simulink model "Final_closeloop_sinus"  (R2024b)
settings: Solver=ode23s  StartTime=0.0  StopTime=150  RelTol=1e-3
libraries: slpidlib x16
(part 2 of 2)

== matlab function Final_closeloop_sinus/M-101 ==
  data: y output; u input
function y  = MX(u) 

% inputs
Q_R = u(1);     % Recycling stream
Q_M = u(2);     % Fresh media stream
C_X_M = u(3);   % Fresh biomass concentration
C_GLU_M = u(4); % Fresh glucose concentration
C_N_M = u(5);   % Fresh nitrogen concentration
C_X_S = u(6);   % Recycle biomass concentration
C_GLU_S = u(7); % Recycle glucose concentration
C_N_S = u(8);   % Recycle nitrogen concentration


% output
y=zeros(4,1);
y(1) = (C_X_S*Q_R+C_X_M*Q_M)/(Q_M+Q_R);         %C_X_F
y(2) = (C_GLU_M*Q_M+C_GLU_S*Q_R)/(Q_M+Q_R);     %C_GLU_F
y(3) = (C_N_M*Q_M+C_N_S*Q_R)/(Q_M+Q_R);         %C_N_F
y(4) = (Q_M+Q_R);                               % Q_F

== matlab function Final_closeloop_sinus/MM-501 ==
  data: y output; u input
function y  = MX(u)

% Inputs: [Q_F, C_mRNA_F, Q_G, C_LNP_G, C_ethanol_G, C_imp1_G, C_imp2_G, C_imp3_G, encapsulation_efficiency]

% Inputs
Q_F = u(1);                                      % Flow rate from Tank F (mRNA solution)
C_mRNA_F = u(2);                                 % mRNA concentration
Q_G = u(3);                                      % Flow rate from Tank G (LNP solution)
C_LNP_G = u(4);                                  % LNP concentration (Tank G)
C_ethanol_G = u(5);                              % Ethanol concentration
C_sucrose_G = u(6);                              % Sucrose concentration
C_imp1_G = u(7);                                 % Impurity 1 concentration 
C_imp2_G = u(8);                                 % Impurity 2 concentration

y = zeros(7, 1);

y(1) = (C_mRNA_F * Q_F)/(Q_F + Q_G);       % Encapsulated mRNA-LNP (assumed 100% encapsulated)
y(2) = (C_LNP_G * Q_F)/(Q_F + Q_G);       % Encapsulated LNP (assumed 100% encapsulated)
y(3) = (C_ethanol_G* Q_G) / (Q_F + Q_G);         % C_ethanol
y(4) = (C_sucrose_G* Q_G) / (Q_F + Q_G);         % C_ethanol
y(5) = (C_imp1_G * Q_G) / (Q_F + Q_G);           % C_Impurity 1
y(6) = (C_imp2_G * Q_G) / (Q_F + Q_G);           % C_Impurity 2
y(7) = (Q_F + Q_G);                                % Total flow rate

end

== matlab function Final_closeloop_sinus/NF-501 ==
  data: u input; y output
function y = NF(u)
%% parameters for nanofiltration 
% a DOW NF90 nanofiltration membrane has been chosen. This type of membrane
% has been used in pharmaceutical applications for API filtrations (title
% reference: Removal of antibiotics from a model wastewater by RO/NF membranes)
%A=0.398443840087261; %membrane surface area [m^2] 
%% parameters for nanofiltration 
%A=0.3984033;
Jw=57.90; %permeate flowrate at 8 bar pressure [l/m^2/h]
Res=Jw/8; %[l/m^2/h/bar]function y  = NN(u)


%input
C_mRNALNP_4=u(1);
C_LNP_4=u(2);
C_Ethanol_4=u(3);
C_Sucrose_4=u(4);
C_IMP1_4=u(5);
C_IMP2_4=u(6);
Q_IN=u(7);
P=u(8);
A=u(9);

tlim=1;
dim=14;
y=zeros(dim,1);


%% Rejection coefficients for different species
Rej=[0.00002*P^4 - 0.0018*P^3 + 0.0145*P^2 + 0.0849*P + 0.22248; 0.01; 0.01; 0.00002*P^4 - 0.0018*P^3 + 0.0145*P^2 + 0.0849*P + 0.22248; 0.01; 0.99];


%% Output calculations

     y(1)=A*Res*P;%permeate volumetric flowrate [l/h];(ref: Continuous purification of
    %active pharmaceutical ingredients using multistage organic solvent nanofiltration membrane cascade)
    y(2)=Q_IN-y(1); %balance on centrifugation+filtration
    

%% Species balances for retentate stream (calculated based on inflow and rejection)
    y(3)=(Q_IN*C_mRNALNP_4)/(y(2)+y(1)*(1-Rej(1)));         % mRNA-LNP concentration in retentate stream
    y(4)=(Q_IN*C_LNP_4)/(y(2)+y(1)*(1-Rej(2)));         % LNP concentration in retentate stream
    y(5)=(Q_IN*C_Ethanol_4)/(y(2)+y(1)*(1-Rej(3)));         % Ethanol concentration in retentate stream
    y(6)=(Q_IN*C_Sucrose_4)/(y(2)+y(1)*(1-Rej(4)));         % Sucrose concentration in retentate stream
    y(7)=(Q_IN*C_IMP1_4)/(y(2)+y(1)*(1-Rej(5)));            % Impurity 1 concentration in retentate stream
    y(8)=(Q_IN*C_IMP2_4)/(y(2)+y(1)*(1-Rej(6)));            % Impurity 2 concentration in retentate stream
   
 %% Species concentrations in permeate stream (calculated based on rejection)
    y(9)=y(3)*(1-Rej(1));                                   % mRNA-LNP concentration in permeate stream
    y(10)=y(4)*(1-Rej(2));                                   % LNP concentration in permeate stream
    y(11)=y(5)*(1-Rej(3));                                   % Ethanol concentration in permeate stream
    y(12)=y(6)*(1-Rej(4));                                  % Sucrose concentration in permeate stream
    y(13)=y(7)*(1-Rej(5));                                  % Impurity 1 concentration in permeate stream
    y(14)=y(8)*(1-Rej(6));                                  % Impurity 2 concentration in permeate stream
  

end

== matlab function Final_closeloop_sinus/VSP-503 ==
  data: u input size=2; y output size=2
function y  = Pump(u)

%input
Q_C=u(1);
n=u(2);


y=zeros(2,1);

% output

y(1)=Q_C;
y(2)=((-0.085*Q_C^2 - 0.0000329*Q_C*n + 0.0000155555555555556*n^2)*(997*9.81))/10^5;


end

== matlab function Final_closeloop_sinus/MATLAB Function1 ==
  data: u input; y output
function y = Formulation_medium(u)
    % Inputs
    Q = u(1);                                   % Total flow rate (L/h)
    C_mRNA = u(2);                              % Concentration of mRNA (g/L)

    % Distribution of flow rates
    Q_Ethanol = Q/3;                            % Ethanol flow (1/3 of total flow)
    Q_LNP = Q / 3;                              % LNP flow (1/3 of total flow)
    Q_Sucrose = Q*10;                            % LNP flow (1/3 of total flow)

    % Concentrations
    C_LNP = C_mRNA / 0.029;                     % LNP concentration (g/g)
    C_Sucrose = Q_Sucrose *0.1;                   % Sucrose concentration
    C_Impurities_1 = Q_Ethanol * 0.05;          % Impurity 1: 5% of ethanol flow
    C_Impurities_2 = Q_Ethanol * 0.05;          % Impurity 2: 5% of ethanol flow

    % Outputs
    y = zeros(1, 6); % Output vector
    y(1) = (Q_Ethanol + Q_LNP + Q_Sucrose);       % Total flow rate (ethanol + LNP)
    y(2) = (C_LNP * Q_LNP) / y(1);              % Weighted concentration of LNP
    y(3) = (Q_Ethanol) / y(1);        % Weighted Ethanol concentration
    y(4) = (C_Sucrose*Q_Sucrose) / y(1);        % Weighted Sucrose concentration
    y(5) = (C_Impurities_1 * Q_Ethanol) / y(1); % Weighted concentration of Impurity 1
    y(6) = (C_Impurities_2 * Q_Ethanol) / y(1); % Weighted concentration of Impurity 2
end

== matlab function Final_closeloop_sinus/MATLAB Function3 ==
  data: u input; y output
function y = Membrane_area(u)
    % Inputs
    Q_IN = u(1);  % Total flow rate (L/h)
    P = u(2);     % Pressure (kPa)

    % Parameters for nanofiltration
    P_0 = 0.49;        % Reference pressure (kPa)
    alpha_0 = 10.2 * 10^12; % Reference alpha (kPa*s)^-1
    n = 0.5;            % Exponent for alpha
    eta_perm = 1.0 * 10^-8;  % Viscosity (kPa*s)
    m_x_c = 7.7 * 10^-3;    % Membrane permeability coefficient (kg)
    R_m = 1.26 * 10^12;     % Membrane resistance (1/m)

    % Calculate alpha based on the pressure
    alpha = alpha_0 * (P / P_0)^n;

    % Desired permeate flow is 40% of Q_IN
    desired_permeate_flow = 0.8 * Q_IN;

    % Initial guess for membrane area A (in m^2)
    A_min = 1e-6;   % Min value for area (to avoid division by zero)
    A_max = 10;     % Max value for area (arbitrary large number)
    tolerance = 1e-6;  % Tolerance for solution accuracy
    max_iter = 100;  % Maximum number of iterations

    % Bisection method to find A
    for iter = 1:max_iter
        A_mid = (A_min + A_max) / 2;
        
        % Calculate R_C based on A_mid
        R_C_mid = alpha * m_x_c / A_mid;

        % Calculate permeate flow based on A_mid
        permeate_flow = (P / (eta_perm * (R_m + R_C_mid))) * A_mid * 1000 * 3600;

        % Check if the calculated permeate flow is close to the desired value
        if abs(permeate_flow - desired_permeate_flow) < tolerance
            break;
        elseif permeate_flow > desired_permeate_flow
            A_max = A_mid;  % Search in the lower half
        else
            A_min = A_mid;  % Search in the upper half
        end
    end

    % The solution found for A is stored in A_mid
    A_value = A_mid;

    % Output the membrane area (in m^2)
    y = A_value;  % Membrane area (m^2)
end

== matlab function Final_closeloop_sinus/MATLAB Function6 ==
  data: u input; y output
function y = Membrane_area(u)
    % Inputs
    Q_IN = u(1);                    % Total flow rate (L/h)
    P = u(2);                       % Pressure (kPa)

    % Parameters for nanofiltration
    P_0 = 0.49;                     % Reference pressure (kPa)
    alpha_0 = 10.2 * 10^12;         % Reference alpha (kPa*s)^-1
    n = 0.5;                        % Exponent for alpha
    eta_perm = 1.0 * 10^-8;         % Viscosity (kPa*s)
    m_x_c = 7.7 * 10^-3;            % Membrane permeability coefficient (kg)
    R_m = 1.26 * 10^12;             % Membrane resistance (1/m)

    % Calculate alpha based on the pressure
    alpha = alpha_0 * (P / P_0)^n;

    % Desired permeate flow is 80% of Q_IN
    desired_permeate_flow = 0.8 * Q_IN;

    % Initial guess for membrane area A (in m^2)
    A_min = 1e-6;                   % Min value for area (to avoid division by zero)
    A_max = 10;                     % Max value for area (arbitrary large number)
    tolerance = 1e-6;               % Tolerance for solution accuracy
    max_iter = 100;                 % Maximum number of iterations

    % Bisection method to find A
    for iter = 1:max_iter
        A_mid = (A_min + A_max) / 2;
        
        % Calculate R_C based on A_mid
        R_C_mid = alpha * m_x_c / A_mid;

        % Calculate permeate flow based on A_mid
        permeate_flow = (P / (eta_perm * (R_m + R_C_mid))) * A_mid * 1000 * 3600;

        % Check if the calculated permeate flow is close to the desired value
        if abs(permeate_flow - desired_permeate_flow) < tolerance
            break;
        elseif permeate_flow > desired_permeate_flow
            A_max = A_mid;          % Search in the lower half
        else
            A_min = A_mid;          % Search in the upper half
        end
    end

    % The solution found for A is stored in A_mid
    A_value = A_mid;

    % Output the membrane area (in m^2)
    y = A_value;                    % Membrane area (m^2)
end

== matlab function Final_closeloop_sinus/MF-501 ==
  data: u input; y output
function y  = MF(u)

%input
C_mRNALNP_4=u(1);
C_sucrose_4=u(2);
C_IMP2_4=u(3);
Q_IN=u(4);
P=u(5);
A=u(6);

%% parameters for microfiltration 

%A=0.00045; %m^2
Jw=800;                 % Permeate flowrate at 1.4 bar pressure [l/m^2/h]
Res=Jw/P;               % [l/m^2/h/bar]function y  = NN(u)

tlim=1;                 % h
dim=8;
y=zeros(dim,1);


%% Rejection coefficients for different species
Rej=[0.01; 0.01; -0.048272*P^4-0.035917*P^3+0.087656*P^2+0.49559*P+0.40839];

%% Output calculations

    y(1)=A*Res*P;       % permeate volumetric flowrate [l/h];(ref: Continuous purification of active pharmaceutical ingredients using multistage organic solvent nanofiltration membrane cascade)
    y(2)=Q_IN-y(1);     % balance on centrifugation+filtration
    
%% Species balances for retentate stream (calculated based on inflow and rejection)
    y(3)=(Q_IN*C_mRNALNP_4)/(y(2)+y(1)*(1-Rej(1)));         % mRNA-LNP in retentate stream
    y(4)=(Q_IN*C_sucrose_4)/(y(2)+y(1)*(1-Rej(2)));         % Sucrose in retentate stream
    y(5)=(Q_IN*C_IMP2_4)/(y(2)+y(1)*(1-Rej(3)));            % Impurity 2 in retentate stream
   
 %% Species concentrations in permeate stream (calculated based on rejection)
    y(6)=y(3)*(1-Rej(1));                                   % mRNA-LNP in permeate stream
    y(7)=y(4)*(1-Rej(2));                                   % Sucrose in permeate stream
    y(8)=y(5)*(1-Rej(3));                                   % Impurity 2 permeate
    
end

== matlab function Final_closeloop_sinus/VSP-504 ==
  data: u input size=2; y output size=2
function y  = Pump(u)

%input
Q_C=u(1);
n=u(2);


y=zeros(2,1);

% output

y(1)=Q_C;
y(2)=((-0.085*Q_C^2 - 0.0000329*Q_C*n + 0.0000155555555555556*n^2)*(997*9.81))/10^5;


end

== matlab function Final_closeloop_sinus/MATLAB Function ==
  data: u input; y output
function y = Flow(u)
% Flow Function to calculate the required flow rate for a given concentration
% Inputs:
% u(1) - C1: Original concentration (g/L)
% u(2) - f1: Original flow rate (L/h)
% u(3) - C2: New concentration (g/L)
%
% Output:
% y - f2: Required flow rate (L/h) to achieve the same total mass flow T

% Input assignments
C1 = u(1);  % Original concentration (g/L)
f1 = u(2);  % Original flow rate (L/h)
C2 = u(3);  % New concentration (g/L)

% Calculate the required flow rate f2
y = (C1 * f1) / C2;  % New flow rate to maintain the same total mass flow

% Ensure the output is between 5 and 8
if y < 0.000001
    y = 0.000001;
elseif y > 8
    y = 8;
end

end

== matlab function Final_closeloop_sinus/MATLAB Function14 ==
  data: u input; y output
function y = Membrane_area(u)
    % Inputs
    Q_IN = u(1);  % Total flow rate (L/h)
    P = u(2);     % Pressure (kPa)

    % Parameters for nanofiltration
    P_0 = 0.49;        % Reference pressure (kPa)
    alpha_0 = 10.2 * 10^12; % Reference alpha (kPa*s)^-1
    n = 0.5;            % Exponent for alpha
    eta_perm = 1.0 * 10^-8;  % Viscosity (kPa*s)
    m_x_c = 7.7 * 10^-3;    % Membrane permeability coefficient (kg)
    R_m = 1.26 * 10^12;     % Membrane resistance (1/m)

    % Calculate alpha based on the pressure
    alpha = alpha_0 * (P / P_0)^n;

    % Desired permeate flow is 80% of Q_IN
    desired_permeate_flow = 0.8 * Q_IN;

    % Initial guess for membrane area A (in m^2)
    A_min = 1e-6;   % Min value for area (to avoid division by zero)
    A_max = 10;     % Max value for area (arbitrary large number)
    tolerance = 1e-6;  % Tolerance for solution accuracy
    max_iter = 100;  % Maximum number of iterations

    % Bisection method to find A
    for iter = 1:max_iter
        A_mid = (A_min + A_max) / 2;
        
        % Calculate R_C based on A_mid
        R_C_mid = alpha * m_x_c / A_mid;

        % Calculate permeate flow based on A_mid
        permeate_flow = (P / (eta_perm * (R_m + R_C_mid))) * A_mid * 1000 * 3600;

        % Check if the calculated permeate flow is close to the desired value
        if abs(permeate_flow - desired_permeate_flow) < tolerance
            break;
        elseif permeate_flow > desired_permeate_flow
            A_max = A_mid;  % Search in the lower half
        else
            A_min = A_mid;  % Search in the upper half
        end
    end

    % The solution found for A is stored in A_mid
    A_value = A_mid;

    % Output the membrane area (in m^2)
    y = A_value;  % Membrane area (m^2)
end

== matlab function Final_closeloop_sinus/P ==
  data: u input; y output
function y = Purge(u)

% inputs
Q_R=u(1);
Q_P=u(2);


y=zeros(1,1);
y(1) = Q_R*Q_P; % recycle stream

== matlab function Final_closeloop_sinus/MATLAB Function15 ==
  data: u input; y output
function y = membrane_area(u)
    % Inputs
    Q_IN = u(1);  % Total flow rate (L/h)
    P = u(2);     % Pressure (kPa)

    % Parameters
    Jw = 57.90;       % Permeate flow rate at 8 bar pressure [L/m^2/h]
    Res = Jw / 8;     % Permeability [L/m^2/h/bar]
    desired_permeate_flow = 0.8 * Q_IN; % Desired permeate flow [L/h]

    % Initial bounds for membrane area A (m^2)
    A_min =0.01;  % Minimum possible area
    A_max = 10;    % Arbitrary maximum area
    tolerance = 1e-6;  % Tolerance for convergence
    max_iter = 100;    % Maximum iterations for bisection method

    % Bisection method to find A
    for iter = 1:max_iter
        % Midpoint of current range for A
        A_mid = (A_min + A_max) / 2;

        % Calculate permeate flow using the updated equation
        permeate_flow = A_mid * Res * P; % [L/h]

        % Check convergence
        if abs(permeate_flow - desired_permeate_flow) < tolerance
            break;  % Converged to the solution
        elseif permeate_flow > desired_permeate_flow
            A_max = A_mid;  % Adjust upper bound
        else
            A_min = A_mid;  % Adjust lower bound
        end
    end

    % Output the membrane area
    y = A_mid;  % Membrane area (m^2)
end

== matlab function Final_closeloop_sinus/MATLAB Function18 ==
  data: u input; y output
function y = Membrane_area(u)
    % Inputs
    Q_IN = u(1);  % Total flow rate (L/h)
    P = u(2);     % Pressure (kPa)

    % Parameters
    Jw=800; %permeate flowrate at 1.4 bar pressure [l/m^2/h]
    Res=Jw/P; %[l/m^2/h/bar]function y  = NN(u)
    desired_permeate_flow = 0.8 * Q_IN; % Desired permeate flow [L/h]

    % Initial bounds for membrane area A (m^2)
    A_min =0.1*10e-6;  % Minimum possible area
    A_max = 10;    % Arbitrary maximum area
    tolerance = 1e-6;  % Tolerance for convergence
    max_iter = 100;    % Maximum iterations for bisection method

    % Bisection method to find A
    for iter = 1:max_iter
        % Midpoint of current range for A
        A_mid = (A_min + A_max) / 2;

        % Calculate permeate flow using the updated equation
        permeate_flow = A_mid * Res * P; % [L/h]

        % Check convergence
        if abs(permeate_flow - desired_permeate_flow) < tolerance
            break;  % Converged to the solution
        elseif permeate_flow > desired_permeate_flow
            A_max = A_mid;  % Adjust upper bound
        else
            A_min = A_mid;  % Adjust lower bound
        end
    end

    % Output the membrane area
    y = A_mid;  % Membrane area (m^2)
end

== matlab function Final_closeloop_sinus/MATLAB Function2 ==
  data: u input; y output
function y = Flow(u)
% Flow Function to calculate the required flow rate for a given concentration
% Inputs:
% u(1) - C1: Original concentration (g/L)
% u(2) - f1: Original flow rate (L/h)
% u(3) - C2: New concentration (g/L)
%
% Output:
% y - f2: Required flow rate (L/h) to achieve the same total mass flow T

% Input assignments
C1 = u(1);  % Original concentration (g/L)
f1 = u(2);  % Original flow rate (L/h)
C2 = u(3);  % New concentration (g/L)

% Calculate the required flow rate f2
y = (C1 * f1) / C2;  % New flow rate to maintain the same total mass flow

% Ensure the output is between 5 and 8
if y < 0.000001
    y = 0.000001;
elseif y > 8
    y = 8;
end

end

== matlab function Final_closeloop_sinus/MATLAB Function7 ==
  data: u input; y output
function y = Flow(u)
% Flow Function to calculate the required flow rate for a given concentration
% Inputs:
% u(1) - C1: Original concentration (g/L)
% u(2) - f1: Original flow rate (L/h)
% u(3) - C2: New concentration (g/L)
%
% Output:
% y - f2: Required flow rate (L/h) to achieve the same total mass flow T

% Input assignments
C1 = u(1);  % Original concentration (g/L)
f1 = u(2);  % Original flow rate (L/h)
C2 = u(3);  % New concentration (g/L)

% Calculate the required flow rate f2
y = (C1 * f1) / C2;  % New flow rate to maintain the same total mass flow

% Ensure the output is between 5 and 8
if y < 0.000001
    y = 0.000001;
elseif y > 8
    y = 8;
end

end

== matlab function Final_closeloop_sinus/MATLAB Function10 ==
  data: u input; y output
function y = Flow(u)
% Flow Function to calculate the required flow rate for a given concentration
% Inputs:
% u(1) - C1: Original concentration (g/L)
% u(2) - f1: Original flow rate (L/h)
% u(3) - C2: New concentration (g/L)
%
% Output:
% y - f2: Required flow rate (L/h) to achieve the same total mass flow T

% Input assignments
C1 = u(1);  % Original concentration (g/L)
f1 = u(2);  % Original flow rate (L/h)
C2 = u(3);  % New concentration (g/L)

% Calculate the required flow rate f2
y = (C1 * f1) / C2;  % New flow rate to maintain the same total mass flow

% Ensure the output is between 5 and 8
if y < 0.000001
    y = 0.000001;
elseif y > 8
    y = 8;
end

end

== matlab function Final_closeloop_sinus/UF-101 ==
  data: u input; y output
function y  = UF(u)

%Input
C_X_4=u(1);
C_GLU_4=u(2);
C_N_4=u(3);
Q_IN=u(4);
P=u(5);

%% parameters for nanofiltration 

P_0 = 0.49;              % referece pressure (kPa)
alpha_0=10.2*10^12;      % reference value
n=0.5;                   % 
A=0.014;                 % membrane area (m^2)
eta_perm=1.0*10^-8;      % Viscosity (kPa*s)
m_x_c=7.7*10^-3;         % (kg)
R_m =1.26*10^12;         % (1/m)

% Calculate alpha based on P_TM
alpha = alpha_0 * (P / P_0)^n;

% Calculate R_C
R_C = alpha * (m_x_c) / A;

dim=8;
y=zeros(dim,1);

%% Rejection coefficients for different species
Rej=[-0.0250*P^4-0.0236*P^3+0.0927*P^2+0.4960*P+0.1979; 0.01; 0.01];

%% Output calculation
    y(1)=((P/(eta_perm * (R_m + R_C)))*A)*1000*3600; % Permeate flow (L/m^2/h)

    y(2)=Q_IN-y(1);                                  % Retentate flow

%% Species balances for retentate stream (calculated based on inflow and rejection)
    y(3)=(Q_IN*C_X_4)/(y(2)+y(1)*(1-Rej(1)));        %Biomass species balance retentate stream
    y(4)=(Q_IN*C_GLU_4)/(y(2)+y(1)*(1-Rej(2)));      %Glucose species balance retentate stream
    y(5)=(Q_IN*C_N_4)/(y(2)+y(1)*(1-Rej(3)));        %Nitrogen species balance retentate stream
   
%% Species concentrations in permeate stream (calculated based on rejection)    
    y(6)=y(3)*(1-Rej(1));                            %Biomass concentration in permeate stream
    y(7)=y(4)*(1-Rej(2));                            %Glucose concentration in permeate stream
    y(8)=y(5)*(1-Rej(3));                            %Nitrogen concentration in permeate stream

end

== matlab function Final_closeloop_sinus/MATLAB Function8 ==
  data: value input; y output; t input
function y = test_input(value, t)
% Test Input Function for PID Stability
% This function varies the input to the PID control from 5% below to 5% above
% the given value over time using a sinusoidal pattern.
%
% Inputs:
%   value - The steady-state value to test around
%   t     - Current simulation time
%
% Output:
%   y     - The dynamic input value for the PID

    % Parameters
    amplitude = 0.1 * value;   % Amplitude for 5% variation
    frequency = 0.1;            % Frequency of oscillation (Hz)

    % Calculate the test input as a sinusoidal wave
    y = value + amplitude * sin(2 * pi * frequency * t);
end

== matlab function Final_closeloop_sinus/VSP-101 ==
  data: u input size=2; y output size=2
function y  = Pump(u)

%input
Q_C=u(1);
n=u(2);

dim=2;

y=zeros(dim,1);

% output

y(1)=Q_C;
y(2)=((-0.085*Q_C^2 - 0.0000329*Q_C*n + 0.0000155555555555556*n^2)*(997*9.81))/10^5;


end

== matlab function Final_closeloop_sinus/VSP-204 ==
  data: u input size=2; y output size=2
function y  = Pump(u)

%input
Q_C=u(1);
n=u(2);



y=zeros(2,1);

%output

y(1)=Q_C;
y(2)=((-0.085*Q_C^2 - 0.0000329*Q_C*n + 0.0000155555555555556*n^2)*(997*9.81))/10^5;


end

== matlab function Final_closeloop_sinus/UF-201 ==
  data: u input; y output
function y  = UF(u)

%input
C_X_4=u(1);
C_DIS_4=u(2);
C_PLASMID_4=u(3);
C_DE_4=u(4);
C_ENDO_4=u(5);
C_ALKA_4=u(6);
C_CH3CO2K_4=u(7);
Q_IN=u(8);
P=u(9);
A=u(10);

%% parameters for nanofiltration 

P_0 = 0.49;                     % referece pressure (kPa)
alpha_0=10.2*10^12;             % reference.
n=0.5;                          % 
eta_perm=1.0*10^-8;             % Viscosity (kPa*s)
m_x_c=7.7*10^-3;                % (kg)
R_m =1.26*10^12;                % (1/m)

% Calculate alpha based on P_TM
alpha = alpha_0 * (P / P_0)^n;

% Calculate R_C
R_C = alpha * (m_x_c) / A;


dim=16;
y=zeros(dim,1);

%% Rejection coefficients for different species
Rej=[-0.0250*P^4-0.0236*P^3+0.0927*P^2+0.4960*P+0.1979; -0.0250*P^4-0.0236*P^3+0.0927*P^2+0.4960*P+0.1979; 0.01; 0.01; 0.01; 0.01; 0.01];


%% Output calculation

    y(1)=((P/(eta_perm * (R_m + R_C)))*A)*1000*3600;    % Permeate flow (L/m^2/h)

    y(2)=Q_IN-y(1);                                     % Retentate
    
 %% Species balances for retentate stream (calculated based on inflow and rejection)
    y(3)=(Q_IN*C_X_4)/(y(2)+y(1)*(1-Rej(1)));           % Biomass species balance--retentate stream
    y(4)=(Q_IN*C_DIS_4)/(y(2)+y(1)*(1-Rej(2)));         % Cell disrupts species balance--retentate stream
    y(5)=(Q_IN*C_PLASMID_4)/(y(2)+y(1)*(1-Rej(3)));     % Plasmid species balance--retentate stream
    y(6)=(Q_IN*C_DE_4)/(y(2)+y(1)*(1-Rej(4)));          % Denaturated plasmid species balance--retentate stream
    y(7)=(Q_IN*C_ENDO_4)/(y(2)+y(1)*(1-Rej(5)));        % Endotoxin species balance--retentate stream
    y(8)=(Q_IN*C_ALKA_4)/(y(2)+y(1)*(1-Rej(6)));        % Alkaline buffer species balance--retentate stream
    y(9)=(Q_IN*C_CH3CO2K_4)/(y(2)+y(1)*(1-Rej(7)));     % Neutralization buffer species balance--retentate stream
   
%% Species concentrations in permeate stream (calculated based on rejection)      
    y(10)=y(3)*(1-Rej(1));                              % Biomass concentration in permeate stream
    y(11)=y(4)*(1-Rej(2));                              % Cell disrupt concentration in permeate stream
    y(12)=y(5)*(1-Rej(3));                              % Plasmid concentration in permeate stream
    y(13)=y(6)*(1-Rej(4));                              % Denaturated plasmid concentration in permeate stream
    y(14)=y(7)*(1-Rej(5));                              % Endotoxin concentration in permeate stream
    y(15)=y(8)*(1-Rej(6));                              % Alkaline buffer concentration in permeate stream
    y(16)=y(9)*(1-Rej(7));                              % Neutralization buffer concentration in permeate stream
    

end

== matlab function Final_closeloop_sinus/MATLAB Function4 ==
  data: u input; y output
function y = Resuspension (u)

% inputs
Q=u(1);
C_X_S=u(2);
C_NaOH=u(3);

%reaction
Q_resuspension=Q*10;
Q_Alkaline=Q_resuspension;


y=zeros(1,3);
y(1) = (C_X_S*Q)/(Q+Q_resuspension+Q_Alkaline);             %C_X_F
y(2) = (Q+Q_resuspension+Q_Alkaline);                       %Q total
y(3) = (C_NaOH*Q_Alkaline)/(Q+Q_resuspension+Q_Alkaline);   %NaOH

== matlab function Final_closeloop_sinus/MATLAB Function5 ==
  data: u input; y output
function y = Neutralization(u)

% inputs
Q=u(1);
C_X_S=u(2);
C_Dis=u(3);
C_Plasmid=u(4);
C_De=u(5);
C_Endo=u(6);
C_NaOH=u(7);
C_CH3CO2K=u(8);

% Reaction
Q_neutralization=Q*0.5;

y=zeros(1,8);
y(1) = (Q+Q_neutralization);                                %Q total
y(2) = (C_X_S*Q)/(Q+Q_neutralization);                      %C_X_F
y(3) = (C_Dis*Q)/(Q+Q_neutralization);                      %C_disruption_F
y(4) = (C_Plasmid*Q)/(Q+Q_neutralization);                  %C_plasmid_F
y(5) = (C_De*Q)/(Q+Q_neutralization);                       %C_denaturated_F
y(6) = (C_Endo*Q)/(Q+Q_neutralization);                     %C_endotoxin_F
y(7) = (C_NaOH*Q)/(Q+Q_neutralization);                     %C_NaOH_F
y(8) = (C_CH3CO2K*Q_neutralization)/(Q+Q_neutralization);   %C_CH3CO2K_F

== matlab function Final_closeloop_sinus/UF-301 ==
  data: u input; y output
function y  = UF(u)

%input
C_pDNA=u(1);
C_lin_pDNA=u(2);
C_Impurities=u(3);
C_Enzyme=u(4);
Q_IN=u(5);
P=u(6);
A=u(7);

%% parameters for nanofiltration 

P_0 = 0.49; % referece pressure (kPa)
alpha_0=10.2*10^12; % reference.
n=0.5; % 
%A=0.1036; % membrane area (m^2)
eta_perm=1.0*10^-8; % Viscosity (kPa*s)
m_x_c=7.7*10^-3; % (kg)
R_m =1.26*10^12; % (1/m)

% Calculate alpha based on P_TM
alpha = alpha_0 * (P / P_0)^n;

% Calculate R_C
R_C = alpha * (m_x_c) / A;


dim=10;
y=zeros(dim,1);

 %% Rejection coefficients for different species
Rej=[0.01; 0.01; 0.01; -0.0250*P^4-0.0236*P^3+0.0927*P^2+0.4960*P+0.1979];


%% Output calculation

    y(1)=((P/(eta_perm * (R_m + R_C)))*A)*1000*3600;% Permeate flow (L/m^2/h)

    y(2)=Q_IN-y(1); % Retentate
    
%% Species balances for retentate stream (calculated based on inflow and rejection)
    y(3)=(Q_IN*C_pDNA)/(y(2)+y(1)*(1-Rej(1)));              % pDNA species balance retentate stream
    y(4)=(Q_IN*C_lin_pDNA)/(y(2)+y(1)*(1-Rej(2)));          % LinpDNA species balance retentate stream
    y(5)=(Q_IN*C_Impurities)/(y(2)+y(1)*(1-Rej(3)));        % Impurties species balance retentate stream
    y(6)=(Q_IN*C_Enzyme)/(y(2)+y(1)*(1-Rej(4)));            % Enzyme plasmid species balance retentate stream

%% Species concentrations in permeate stream (calculated based on rejection) 
    y(7)=y(3)*(1-Rej(1));                                   % pDNA concentration in permeate stream
    y(8)=y(4)*(1-Rej(2));                                   % LinpDNA concentration in permeate stream
    y(9)=y(5)*(1-Rej(3));                                   % Impurities concentration in permeate stream
    y(10)=y(6)*(1-Rej(4));                                  % Enzyme concentration in permeate stream

end

== matlab function Final_closeloop_sinus/VSP-301 ==
  data: u input size=2; y output size=2
function y  = Pump(u)

%input
Q_C=u(1);
n=u(2);



y=zeros(2,1);

% output

y(1)=Q_C;
y(2)=((-0.085*Q_C^2 - 0.0000329*Q_C*n + 0.0000155555555555556*n^2)*(997*9.81))/10^5;


end

== matlab function Final_closeloop_sinus/UF-401 ==
  data: u input; y output
function y = UF(u)
    % Input concentrations for each species in the feed stream
    C_mRNA = u(1);              % mRNA concentration (g/L)
    C_impurities = u(2);        % Impurities concentration (g/L)
    C_T7 = u(3);                % Ea T7 concentration (g/L)
    C_linpDNA = u(4);           % linpDNA concentration (g/L)
    C_cleancap = u(5);          % CleanCap concentration (g/L)
    C_magnesium = u(6);         % MgAcetate concentration (g/L)
    C_nucleo = u(7);            % Nucleotides concentration (g/L)
    C_degrade = u(8);           % Degrade concentration (g/L)
    C_Ea_DNase = u(9);          % DNase I concentration (g/L)
    Q_IN = u(10);               % Inflow rate (L/h)
    P = u(11);                  % Transmembrane pressure (kPa)
    A=u(12);

    %% Parameters for nanofiltration
    P_0 = 0.49;           % Reference pressure (kPa)
    alpha_0 = 10.2e12;    % Reference alpha
    n = 0.5;              % Pressure exponent
    eta_perm = 1.0e-8;    % Viscosity (kPa*s)
    m_x_c = 7.7e-3;       % (kg)
    R_m = 1.26e12;        % (1/m)

    % Calculate alpha based on P_TM
    alpha = alpha_0 * (P / P_0)^n;

    % Calculate R_C
    R_C = alpha * (m_x_c) / A;

    % Time and dimension parameters
    dim = 20;           % Number of outputs (8 species in both retentate and permeate)
    y = zeros(dim, 1);  % Initialize output vector

    %% Rejection coefficients for different species
    Rej = [-0.0250*P^4 - 0.0236*P^3 + 0.0927*P^2 + 0.4960*P + 0.1979; 0.50; -0.0250*P^4 - 0.0236*P^3 + 0.0927*P^2 + 0.4960*P + 0.1979; 0.01; -0.0250*P^4 - 0.0236*P^3 + 0.0927*P^2 + 0.4960*P + 0.1979; -0.0250*P^4 - 0.0236*P^3 + 0.0927*P^2 + 0.4960*P + 0.1979; 0.01; 0.01;0.01];
   
    %% Output calculations
    % Permeate flow rate (L/m^2/h)
    y(1) = (P / (eta_perm * (R_m + R_C))) * A * 1000 * 3600;            % Permeate flow (L/m^2/h)
    y(2) = Q_IN - y(1);                                                 % Retentate flow
    
    % Species balances for retentate stream (calculated based on inflow and rejection)
   y(3) = (Q_IN * C_mRNA) / (y(2) + y(1) * (1 - Rej(1)));               % mRNA concentration in retentate
    y(4) = (Q_IN * C_impurities) / (y(2) + y(1) * (1 - Rej(2)));        % Assumed 50% impurities futher in the system.Impurities concentration in retentate
    y(5) = (Q_IN * C_T7) / (y(2) + y(1) * (1 - Rej(3)));                % Ea T7 concentration in retentate
    y(6) = (Q_IN * C_linpDNA) / (y(2) + y(1) * (1 - Rej(4)));           % linpDNA (DNA template) concentration in retentate
    y(7) = (Q_IN * C_cleancap) / (y(2) + y(1) * (1 - Rej(5)));          % CleanCap concentration in retentate
    y(8) = (Q_IN * C_magnesium) / (y(2) + y(1) * (1 - Rej(6)));         % MgAcetate concentration in retentate
    y(9) = (Q_IN * C_nucleo) / (y(2) + y(1) * (1 - Rej(7)));            % Nucleotides concentration in retentate
    y(10) = (Q_IN * C_degrade) / (y(2) + y(1) * (1 - Rej(8)));          % Degrade concentration in retentate
    y(11) = (Q_IN * C_Ea_DNase) / (y(2) + y(1) * (1 - Rej(9)));         % DNase I concentration in retentatem

    %% Species concentrations in permeate stream (calculated based on rejection)
    y(12) = y(3) * (1 - Rej(1));  % mRNA concentration in permeate
    y(13) = y(4) * (1 - Rej(2));  % Impurities concentration in permeate
    y(14) = y(5) * (1 - Rej(3));  % Ea T7 concentration in permeate
    y(15) = y(6) * (1 - Rej(4));  % linpDNA (DNA template) concentration in permeate
    y(16) = y(7) * (1 - Rej(5));  % CleanCap concentration in permeate
    y(17) = y(8) * (1 - Rej(6));  % MgAcetate concentration in permeate
    y(18) = y(9) * (1 - Rej(7));  % Nucleotides concentration in permeate
    y(19) = y(10) * (1 - Rej(8)); % Degrade concentration in permeate
    y(20) = y(11) * (1 - Rej(9)); % DNase concentration in permeate
 


end

== matlab function Final_closeloop_sinus/VSP-401 ==
  data: u input size=2; y output size=2
function y  = Pump(u)

%input
Q_C=u(1);
n=u(2);



y=zeros(2,1);

% output

y(1)=Q_C;
y(2)=((-0.085*Q_C^2 - 0.0000329*Q_C*n + 0.0000155555555555556*n^2)*(997*9.81))/10^5;


end
